simulink model "lab2"  (R2017a)
settings: Solver=VariableStepAuto  StartTime=0.0  StopTime=1.0  RelTol=1e-3
settings Model: Creator=banci002  LastModifiedBy=banci002

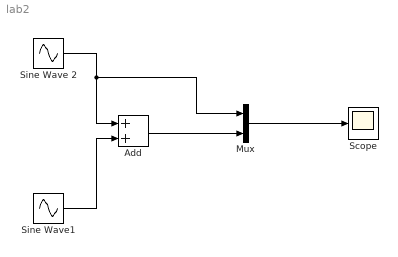
== system lab2 ==
  Add : Sum
  Mux : Mux  Inputs=2
  Scope : Scope
  "Sine Wave 2 " : Sin  Frequency=2*pi*5  Phase=pi  SampleTime=0
  Sine Wave1 : Sin  Frequency=2*pi*5  SampleTime=0
  wires:
  Add/1 -> Mux/2
  Mux/1 -> Scope/1
  Sine Wave1/1 -> Add/2
  "Sine Wave 2 "/1 -> Mux/1, Add/1
